simulink model "basisSL"  (R2015a)
settings: Solver=ode3  StartTime=0.0  StopTime=10.0  RelTol=1e-3
settings Model: Creator=Bryan  LastModifiedBy=Bryan
settings RTWCC: TargetLang=C++
settings GRTTargetCC: MatFileLogging=off  MultiInstanceERTCode=on  CodeInterfacePackaging=C++ class

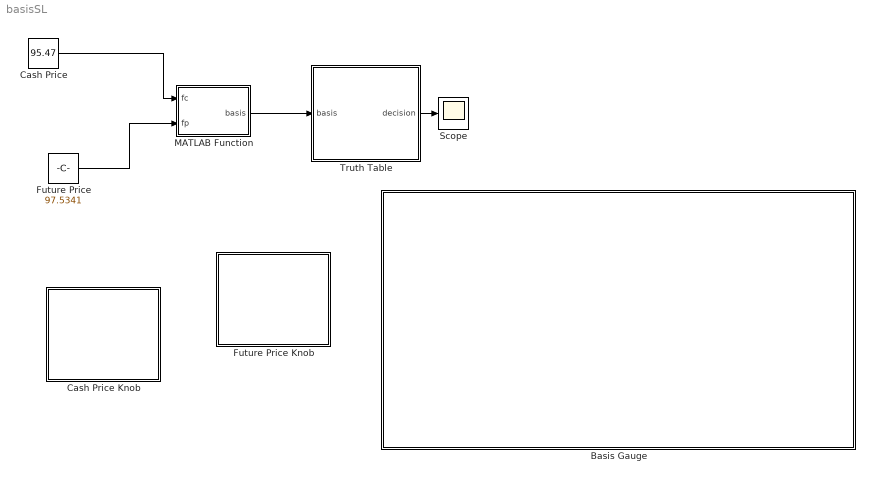
== system basisSL ==
  Basis Gauge : Subsystem  DialogController=hmiCreateDDGDialog  IsWebBlock=on  mask(MathWorksWebBlock){webBlockId=d2efbad3-438b-456a-b27f-2aa1e33f7bba, webBlockType=circulargauge, ShowInLibBrowser=on, ShowInitialText=on, HMISrcModelName=basisSL}
      mask prompts: webBlockId "WebBlock Id"; webBlockType "WebBlock Type"; HMISrcModelName "Source Model"
      mask Help: helpview([docroot '/mapfiles/simulink.map'], 'hmi_gauge')
      mask Display:
      | if strcmp(get_param(bdroot(gcb),'BlockDiagramType'), 'library')
      |     image([(matlabroot) '/toolbox/simulink/hmi/icons/CircularGauge.png']);
      | end
  Cash Price : Constant  Value=95.47
  Cash Price Knob : Subsystem  DialogController=hmiCreateDDGDialog  IsWebBlock=on  mask(MathWorksWebBlock){webBlockId=369989ab-d8f7-45eb-a3b2-571a18cc1d2b, webBlockType=continuousknob, ShowInLibBrowser=on, ShowInitialText=on, HMISrcModelName=basisSL}
      mask prompts: webBlockId "WebBlock Id"; webBlockType "WebBlock Type"; HMISrcModelName "Source Model"
      mask Help: helpview([docroot '/mapfiles/simulink.map'], 'hmi_knob')
      mask Display:
      | if strcmp(get_param(bdroot(gcb),'BlockDiagramType'), 'library')
      |     image([(matlabroot) '/toolbox/simulink/hmi/icons/ContinuousKnob.png']);
      | end
  Future Price : Constant  Value=97.5341
  Future Price Knob : Subsystem  DialogController=hmiCreateDDGDialog  IsWebBlock=on  mask(MathWorksWebBlock){webBlockId=341967c5-d88d-478f-bb67-c676ebabda20, webBlockType=continuousknob, ShowInLibBrowser=on, ShowInitialText=on, HMISrcModelName=basisSL}
      mask prompts: webBlockId "WebBlock Id"; webBlockType "WebBlock Type"; HMISrcModelName "Source Model"
      mask Help: helpview([docroot '/mapfiles/simulink.map'], 'hmi_knob')
      mask Display:
      | if strcmp(get_param(bdroot(gcb),'BlockDiagramType'), 'library')
      |     image([(matlabroot) '/toolbox/simulink/hmi/icons/ContinuousKnob.png']);
      | end
  MATLAB Function : MATLAB Function  TreatAsAtomicUnit=on
  Scope : Scope
  Truth Table : Truth Table  TreatAsAtomicUnit=on
  wires:
  MATLAB Function/1(basis) -> Truth Table/1(basis)
  Truth Table/1(decision) -> Scope/1
  Future Price/1 -> MATLAB Function/2(fp)
  Cash Price/1 -> MATLAB Function/1(fc)

== system basisSL/Basis Gauge ==

== system basisSL/Cash Price Knob ==

== system basisSL/Future Price Knob ==

== matlab function basisSL/Truth Table ==
  data: basis input; decision output
function decision = fcn(basis)

aVarTruthTableCondition_1 = false;
aVarTruthTableCondition_2 = false;


% buy

aVarTruthTableCondition_1 = logical(basis >= 0);

% sell

aVarTruthTableCondition_2 = logical(basis <0);

if (aVarTruthTableCondition_1 && aVarTruthTableCondition_2)
    aFcnTruthTableAction_1();
elseif (~aVarTruthTableCondition_1 && ~aVarTruthTableCondition_2)
    aFcnTruthTableAction_1();
else % Default
    aFcnTruthTableAction_2();
end

function aFcnTruthTableAction_1()

% buy decision

decision = 1;

function aFcnTruthTableAction_2()

% sell

decision = -1;

== matlab function basisSL/MATLAB Function ==
  data: fc input; basis output; fp input
function basis = basisSL(fc,fp)
%#codegen
basis = fc-fp;
